simulink model "PD_Control_Gravity_Compensation"  (R2020b)
settings: Solver=VariableStepAuto  StartTime=0.0  StopTime=10  RelTol=1e-3
undefined symbols (not defined in the file or in its folder): Friction, fwdKine, gravity_load, GravityVector
settings Model: Creator=shra1  LastModifiedBy=punee
settings SFSimCC: CustomCodeUndefinedFunction=UseInterfaceOnly

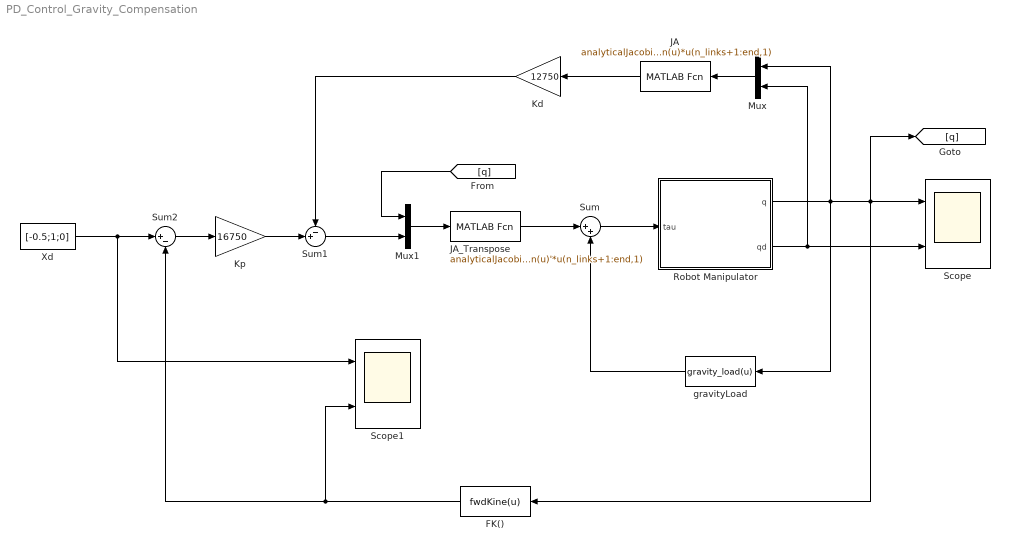
== system PD_Control_Gravity_Compensation ==
  FK() : MATLABFcn  MATLABFcn=fwdKine(u)
  JA : MATLABFcn  MATLABFcn=analyticalJacobian(u)*u(n_links+1:end,1)
  JA_Transpose : MATLABFcn  MATLABFcn=analyticalJacobian(u)'*u(n_links+1:end,1)
  Kd : Gain  Gain=12750
  Kp : Gain  Gain=16750
  Mux : Mux  Inputs=2
  Mux1 : Mux  Inputs=2
  Robot Manipulator : Subsystem
  Scope : Scope  NumInputPorts=2
  Scope1 : Scope  NumInputPorts=2
  Sum : Sum  Inputs=|++
  Sum1 : Sum  Inputs=-+|
  Sum2 : Sum  Inputs=|+-
  Xd : Constant  Value=[-0.5;1;0]
  "gravityLoad " : MATLABFcn  MATLABFcn=gravity_load(u)
  wires:
  JA/1 -> Kd/1
  Robot Manipulator/1(q) -> Mux/1, "gravityLoad "/1, FK()/1, [q], Scope/1
  Robot Manipulator/2(qd) -> Mux/2, Scope/2
  Sum/1 -> Robot Manipulator/1(tau)
  "gravityLoad "/1 -> Sum/2
  JA_Transpose/1 -> Sum/1
  [q] -> Mux1/1
  Sum1/1 -> Mux1/2
  Kd/1 -> Sum1/1
  Kp/1 -> Sum1/2
  Sum2/1 -> Kp/1
  FK()/1 -> Scope1/2, Sum2/2
  Mux/1 -> JA/1
  Mux1/1 -> JA_Transpose/1
  Xd/1 -> Scope1/1, Sum2/1

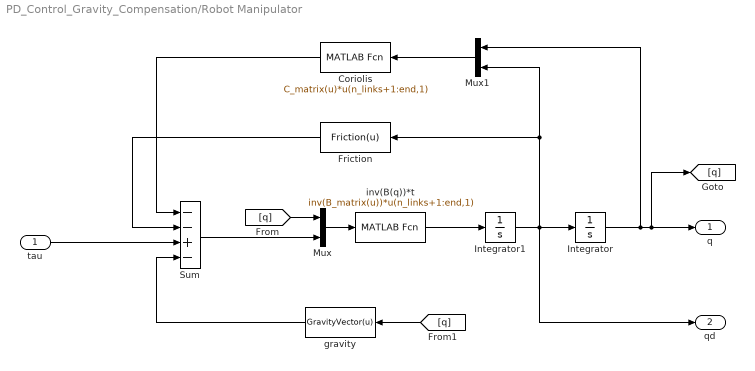
== system PD_Control_Gravity_Compensation/Robot Manipulator ==
  tau : Inport
  Coriolis : MATLABFcn  MATLABFcn=C_matrix(u)*u(n_links+1:end,1)
  Friction : MATLABFcn  MATLABFcn=Friction(u)
  Integrator : Integrator  InitialCondition=[pi/3; -pi/3 ;0]
  Integrator1 : Integrator  InitialCondition=[0;0;0]
  Mux : Mux  Inputs=2
  Mux1 : Mux  Inputs=2
  Sum : Sum  Inputs=--+-  InputSameDT=on  SaturateOnIntegerOverflow=on  OutDataTypeStr=Inherit: Same as first input
  gravity : MATLABFcn  MATLABFcn=GravityVector(u)
  inv(B(q))*t : MATLABFcn  MATLABFcn=inv(B_matrix(u))*u(n_links+1:end,1)
  q : Outport  VectorParamsAs1DForOutWhenUnconnected=off
  qd : Outport  Port=2  VectorParamsAs1DForOutWhenUnconnected=off
  wires:
  Integrator1/1 -> Friction/1, Mux1/2, qd/1, Integrator/1
  inv(B(q))*t/1 -> Integrator1/1
  Mux/1 -> inv(B(q))*t/1
  [q] -> Mux/1
  Integrator/1 -> Mux1/1, [q], q/1
  tau/1 -> Sum/3
  Mux1/1 -> Coriolis/1
  [q] -> gravity/1
  gravity/1 -> Sum/4
  Coriolis/1 -> Sum/1
  Sum/1 -> Mux/2
  Friction/1 -> Sum/2
